simulink model "ECmodel1"  (R2014a)
settings: Solver=ode3  StartTime=0.0  StopTime=6000  FixedStep=10  MaxStep=10  MinStep=10  RelTol=1e-3
settings Model: Creator=Suda  LastModifiedBy=杰

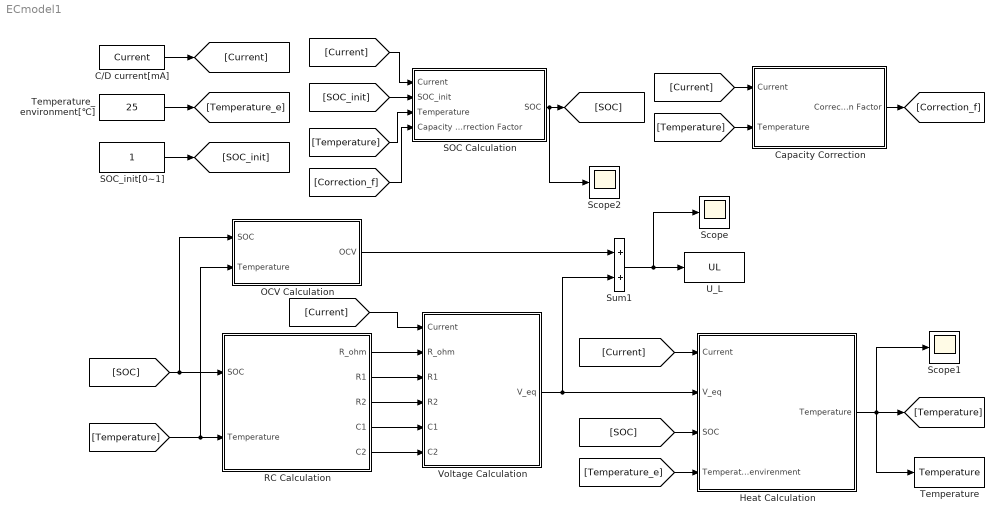
== system ECmodel1 ==
  C/D current[mA] : FromWorkspace  VariableName=Current  SampleTime=0
  Capacity Correction : Subsystem
  Heat Calculation : Subsystem
  OCV Calculation : Subsystem
  RC Calculation : Subsystem
  SOC Calculation : Subsystem
  SOC_init[0~1] : Constant
  Scope : Scope
  Scope1 : Scope
  Scope2 : Scope
      settings: SaveName=ScopeData2
  Sum1 : Sum
  Temperature : ToWorkspace  VariableName=Temperature  SaveFormat=Structure With Time  SampleTime=-1
  Temperature_environment[℃] : Constant  Value=25
  U_L : ToWorkspace  VariableName=UL  SaveFormat=Structure With Time  SampleTime=-1
  Voltage Calculation : Subsystem
  wires:
  OCV Calculation/1(OCV) -> Sum1/1
  RC Calculation/1(R_ohm) -> Voltage Calculation/2("R_ohm ")
  RC Calculation/2(R1) -> Voltage Calculation/3(R1)
  RC Calculation/3(R2) -> Voltage Calculation/4(R2)
  RC Calculation/4(C1) -> Voltage Calculation/5(C1)
  RC Calculation/5(C2) -> Voltage Calculation/6(C2)
  Voltage Calculation/1(V_eq) -> Heat Calculation/2(V_eq), Sum1/2
  Sum1/1 -> Scope/1, U_L/1
  C/D current[mA]/1 -> [Current]
  [Current] -> SOC Calculation/1(Current)
  Temperature_environment[℃]/1 -> [Temperature_e]
  [Temperature] -> SOC Calculation/3("Temperature ")
  SOC Calculation/1(SOC) -> Scope2/1, [SOC]
  [Temperature] -> OCV Calculation/2(Temperature), RC Calculation/2(Temperature)
  [Current] -> Voltage Calculation/1(Current)
  [SOC] -> RC Calculation/1(SOC), OCV Calculation/1(SOC)
  SOC_init[0~1]/1 -> [SOC_init]
  [SOC_init] -> SOC Calculation/2(SOC_init)
  [Temperature_e] -> Heat Calculation/4(Temperature_envirenment)
  [Current] -> Heat Calculation/1(Current)
  Heat Calculation/1(Temperature) -> Temperature/1, Scope1/1, [Temperature]
  [SOC] -> Heat Calculation/3(SOC)
  [Current] -> Capacity Correction/1(Current)
  [Temperature] -> Capacity Correction/2(Temperature)
  [Correction_f] -> SOC Calculation/4(Capacity Correction Factor)
  Capacity Correction/1(" Correction Factor") -> [Correction_f]

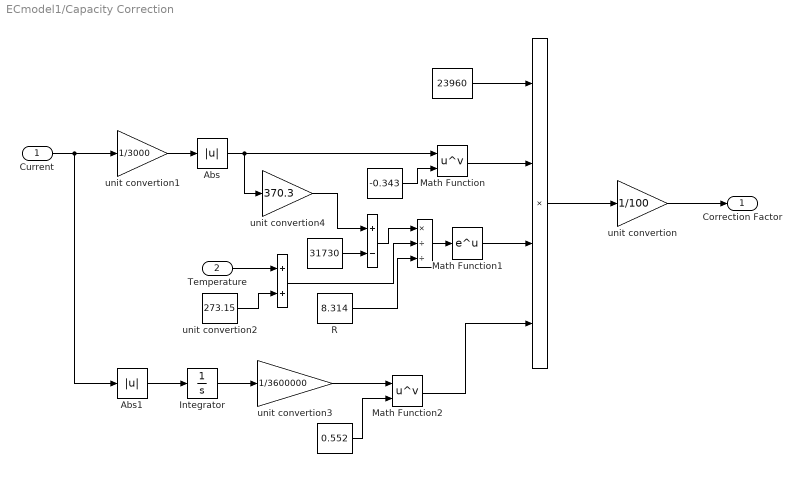
== system ECmodel1/Capacity Correction ==
  Current : Inport
  Temperature : Inport  Port=2
  "  " : Product  Inputs=4
  "     " : Constant  Value=-0.343
  "      " : Constant  Value=23960
  "       " : Constant  Value=31730
  "         " : Sum  Inputs=+-
  "            " : Product  Inputs=*//
  "              " : Sum
  "                 " : Constant  Value=0.552
  Abs : Abs
  Abs1 : Abs
  Integrator : Integrator
  Math Function : Math  Operator=pow  SaturateOnIntegerOverflow=on
  Math Function1 : Math  SaturateOnIntegerOverflow=on
  Math Function2 : Math  Operator=pow  SaturateOnIntegerOverflow=on
  R : Constant  Value=8.314
  unit convertion : Gain  Gain=1/100
  unit convertion1 : Gain  Gain=1/3000
  unit convertion2 : Constant  Value=273.15
  unit convertion3 : Gain  Gain=1/3600000
  unit convertion4 : Gain  Gain=370.3
  " Correction Factor" : Outport
  wires:
  Current/1 -> Abs1/1, unit convertion1/1
  unit convertion1/1 -> Abs/1
  "  "/1 -> unit convertion/1
  "      "/1 -> "  "/1
  Abs/1 -> unit convertion4/1, Math Function/1
  "     "/1 -> Math Function/2
  Math Function/1 -> "  "/2
  Temperature/1 -> "              "/1
  unit convertion2/1 -> "              "/2
  "         "/1 -> "            "/1
  "              "/1 -> "            "/2
  R/1 -> "            "/3
  "            "/1 -> Math Function1/1
  Math Function1/1 -> "  "/3
  Abs1/1 -> Integrator/1
  Integrator/1 -> unit convertion3/1
  "                 "/1 -> Math Function2/2
  Math Function2/1 -> "  "/4
  unit convertion4/1 -> "         "/1
  "       "/1 -> "         "/2
  unit convertion/1 -> " Correction Factor"/1
  unit convertion3/1 -> Math Function2/1

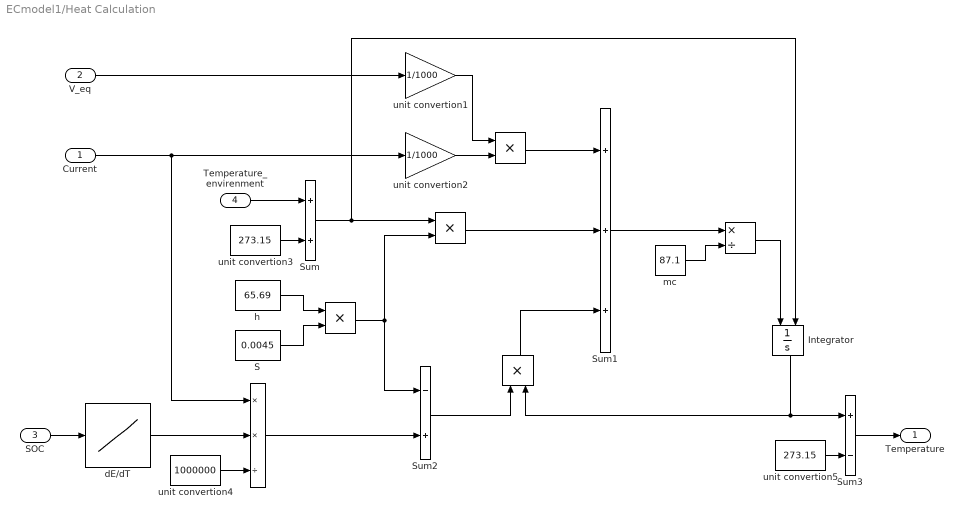
== system ECmodel1/Heat Calculation ==
  Current : Inport
  V_eq : Inport  Port=2
  SOC : Inport  Port=3
  Temperature_envirenment : Inport  Port=4
  "    " : Product
  "     " : Product
  "      " : Product  Inputs=**/
  "       " : Product
  "        " : Product  Inputs=*/
  "                 " : Product
  Integrator : Integrator  InitialConditionSource=external  InitialCondition=273.15
  S : Constant  Value=0.0045
  Sum : Sum
  Sum1 : Sum  Inputs=+++
  Sum2 : Sum  Inputs=-+
  Sum3 : Sum  Inputs=+-
  dE/dT : Lookup_n-D  NumberOfTableDimensions=1  BreakpointsForDimension1=[0.0017,0.0922,0.1907,0.2864,0.3863,0.4883,0.5783,0.6797,0.7686,0.8744,0.9685]  Table=[-0.2986,-0.2442,-0.1088,-0.0392,0.0456,0.0709,0.1089,0.1152,0.0482,0.057,0.1331]  InternalRulePriority=Speed  RndMeth=Simplest  InputSameDT=on
  h : Constant  Value=65.69
  mc : Constant  Value=87.1
  unit convertion1 : Gain  Gain=1/1000
  unit convertion2 : Gain  Gain=1/1000
  unit convertion3 : Constant  Value=273.15
  unit convertion4 : Constant  Value=1000000
  unit convertion5 : Constant  Value=273.15
  Temperature : Outport
  wires:
  V_eq/1 -> unit convertion1/1
  Current/1 -> unit convertion2/1, "      "/1
  unit convertion1/1 -> "    "/1
  unit convertion2/1 -> "    "/2
  Temperature_envirenment/1 -> Sum/1
  unit convertion3/1 -> Sum/2
  h/1 -> "     "/1
  S/1 -> "     "/2
  Sum/1 -> Integrator/2, "       "/1
  "     "/1 -> Sum2/1, "       "/2
  SOC/1 -> dE/dT/1
  dE/dT/1 -> "      "/2
  unit convertion4/1 -> "      "/3
  "      "/1 -> Sum2/2
  unit convertion5/1 -> Sum3/2
  "    "/1 -> Sum1/1
  "       "/1 -> Sum1/2
  Sum2/1 -> "                 "/1
  "                 "/1 -> Sum1/3
  Sum1/1 -> "        "/1
  mc/1 -> "        "/2
  "        "/1 -> Integrator/1
  Integrator/1 -> "                 "/2, Sum3/1
  Sum3/1 -> Temperature/1

== system ECmodel1/OCV Calculation ==
  SOC : Inport
  Temperature : Inport  Port=2
  -10℃ : Subsystem
  10℃ : Subsystem
  25℃ : Subsystem
  40℃ : Subsystem
  55℃ : Subsystem
  Chart : Stateflow chart  TreatAsAtomicUnit=on
  OCV : Outport
  wires:
  SOC/1 -> 55℃/1(SOC), 40℃/1(SOC), 25℃/1(SOC), 10℃/1(SOC), -10℃/1(SOC)
  Temperature/1 -> Chart/1(T)
  -10℃/1(OCV_-10) -> Chart/2(OCV_N10)
  10℃/1(OCV_10) -> Chart/3(OCV_10)
  25℃/1(OCV_25) -> Chart/4(OCV_25)
  40℃/1(OCV_40) -> Chart/5(OCV_40)
  55℃/1(OCV_55) -> Chart/6(OCV_55)
  Chart/1(OCV) -> OCV/1

== system ECmodel1/RC Calculation ==
  SOC : Inport
  Temperature : Inport  Port=2
  Subsystem : Subsystem
  Subsystem1 : Subsystem
  Subsystem2 : Subsystem
  Subsystem3 : Subsystem
  Subsystem4 : Subsystem
  R_ohm : Outport
  R1 : Outport  Port=2
  R2 : Outport  Port=3
  C1 : Outport  Port=4
  C2 : Outport  Port=5
  wires:
  Temperature/1 -> Subsystem4/1(Tempearture), Subsystem3/1(Temperature), Subsystem2/1(Temperature), Subsystem1/1(Tempearture), Subsystem/2(Temperature)
  Subsystem/1(R_ohm) -> R_ohm/1
  Subsystem1/1(R1) -> R1/1
  Subsystem2/1(C1) -> C1/1
  Subsystem3/1(R2) -> R2/1
  Subsystem4/1(C2) -> C2/1
  SOC/1 -> Subsystem/1(SOC)

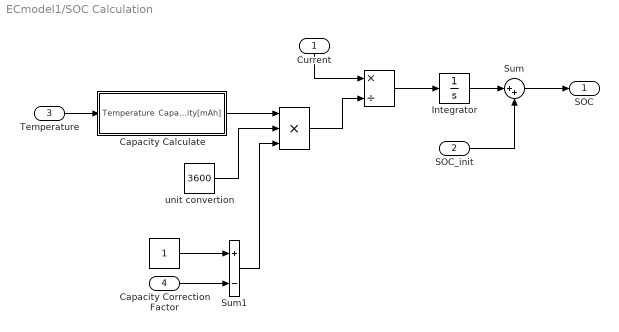
== system ECmodel1/SOC Calculation ==
  Current : Inport
  SOC_init : Inport  Port=2
  "Temperature " : Inport  Port=3
  Capacity Correction Factor : Inport  Port=4
  " " : Constant
  "  " : Product  Inputs=*/
  "    " : Product  Inputs=3
  Capacity Calculate : Subsystem
  Integrator : Integrator
  Sum : Sum  Inputs=|++
  Sum1 : Sum  Inputs=+-
  unit convertion : Constant  Value=3600
  SOC : Outport
  wires:
  "Temperature "/1 -> Capacity Calculate/1(Temperature)
  "    "/1 -> "  "/2
  Integrator/1 -> Sum/1
  SOC_init/1 -> Sum/2
  "  "/1 -> Integrator/1
  Current/1 -> "  "/1
  Capacity Calculate/1(Capacity[mAh]) -> "    "/1
  unit convertion/1 -> "    "/2
  Sum/1 -> SOC/1
  " "/1 -> Sum1/1
  Capacity Correction Factor/1 -> Sum1/2
  Sum1/1 -> "    "/3

== system ECmodel1/Voltage Calculation ==
  Current : Inport
  "R_ohm " : Inport  Port=2
  R1 : Inport  Port=3
  R2 : Inport  Port=4
  C1 : Inport  Port=5
  C2 : Inport  Port=6
  Product : Product
  Subsystem : Subsystem
  Subsystem1 : Subsystem
  Sum : Sum  Inputs=+++
  V_eq : Outport
  wires:
  "R_ohm "/1 -> Product/1
  Product/1 -> Sum/1
  Sum/1 -> V_eq/1
  Current/1 -> Subsystem1/2(Current), Subsystem/2(Current), Product/2
  C1/1 -> Subsystem/1(C1)
  R1/1 -> Subsystem/3(R1)
  Subsystem/1(V1) -> Sum/2
  C2/1 -> Subsystem1/1(C2)
  R2/1 -> Subsystem1/3(R2)
  Subsystem1/1(V2) -> Sum/3

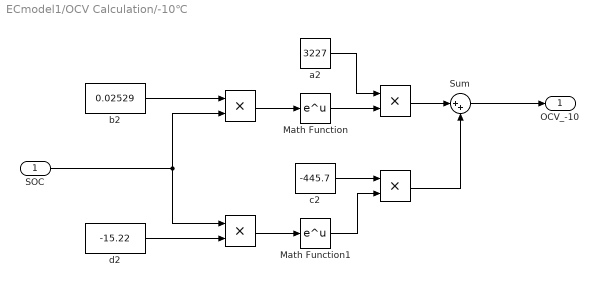
== system ECmodel1/OCV Calculation/-10℃ ==
  SOC : Inport
  " " : Product
  "  " : Product
  "   " : Product
  "    " : Product
  Math Function : Math  SaturateOnIntegerOverflow=on
  Math Function1 : Math  SaturateOnIntegerOverflow=on
  Sum : Sum  Inputs=|++
  a2 : Constant  Value=3227
  b2 : Constant  Value=0.02529
  c2 : Constant  Value=-445.7
  d2 : Constant  Value=-15.22
  OCV_-10 : Outport
  wires:
  Sum/1 -> OCV_-10/1
  d2/1 -> "  "/2
  SOC/1 -> " "/2, "  "/1
  " "/1 -> Math Function/1
  Math Function1/1 -> "    "/2
  "  "/1 -> Math Function1/1
  Math Function/1 -> "   "/2
  c2/1 -> "    "/1
  "   "/1 -> Sum/1
  "    "/1 -> Sum/2
  b2/1 -> " "/1
  a2/1 -> "   "/1

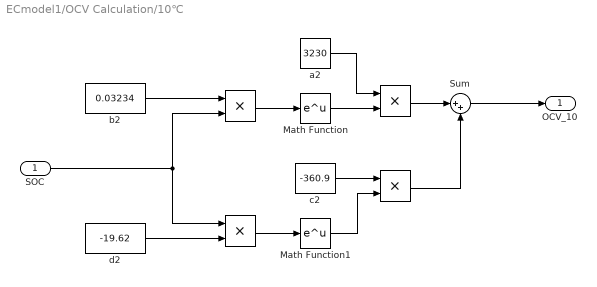
== system ECmodel1/OCV Calculation/10℃ ==
  SOC : Inport
  " " : Product
  "  " : Product
  "   " : Product
  "    " : Product
  Math Function : Math  SaturateOnIntegerOverflow=on
  Math Function1 : Math  SaturateOnIntegerOverflow=on
  Sum : Sum  Inputs=|++
  a2 : Constant  Value=3230
  b2 : Constant  Value=0.03234
  c2 : Constant  Value=-360.9
  d2 : Constant  Value=-19.62
  OCV_10 : Outport
  wires:
  Sum/1 -> OCV_10/1
  d2/1 -> "  "/2
  SOC/1 -> " "/2, "  "/1
  " "/1 -> Math Function/1
  Math Function1/1 -> "    "/2
  "  "/1 -> Math Function1/1
  Math Function/1 -> "   "/2
  c2/1 -> "    "/1
  "   "/1 -> Sum/1
  "    "/1 -> Sum/2
  b2/1 -> " "/1
  a2/1 -> "   "/1

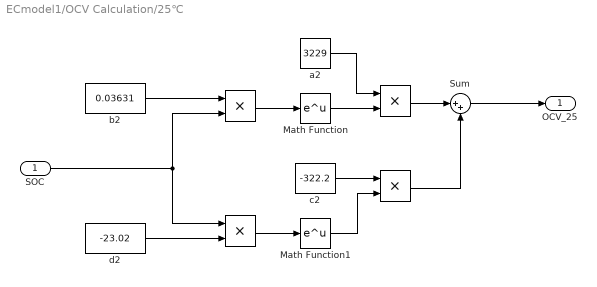
== system ECmodel1/OCV Calculation/25℃ ==
  SOC : Inport
  " " : Product
  "  " : Product
  "   " : Product
  "    " : Product
  Math Function : Math  SaturateOnIntegerOverflow=on
  Math Function1 : Math  SaturateOnIntegerOverflow=on
  Sum : Sum  Inputs=|++
  a2 : Constant  Value=3229
  b2 : Constant  Value=0.03631
  c2 : Constant  Value=-322.2
  d2 : Constant  Value=-23.02
  OCV_25 : Outport
  wires:
  Sum/1 -> OCV_25/1
  d2/1 -> "  "/2
  SOC/1 -> " "/2, "  "/1
  " "/1 -> Math Function/1
  Math Function1/1 -> "    "/2
  "  "/1 -> Math Function1/1
  Math Function/1 -> "   "/2
  c2/1 -> "    "/1
  "   "/1 -> Sum/1
  "    "/1 -> Sum/2
  b2/1 -> " "/1
  a2/1 -> "   "/1

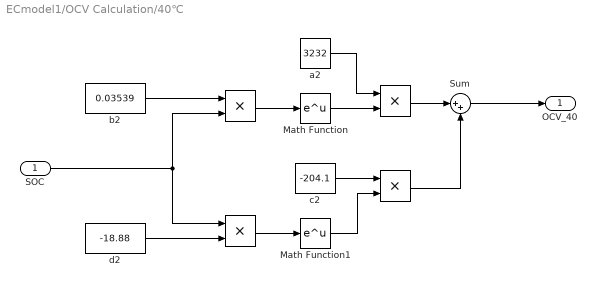
== system ECmodel1/OCV Calculation/40℃ ==
  SOC : Inport
  " " : Product
  "  " : Product
  "   " : Product
  "    " : Product
  Math Function : Math  SaturateOnIntegerOverflow=on
  Math Function1 : Math  SaturateOnIntegerOverflow=on
  Sum : Sum  Inputs=|++
  a2 : Constant  Value=3232
  b2 : Constant  Value=0.03539
  c2 : Constant  Value=-204.1
  d2 : Constant  Value=-18.88
  OCV_40 : Outport
  wires:
  Sum/1 -> OCV_40/1
  d2/1 -> "  "/2
  SOC/1 -> " "/2, "  "/1
  " "/1 -> Math Function/1
  Math Function1/1 -> "    "/2
  "  "/1 -> Math Function1/1
  Math Function/1 -> "   "/2
  c2/1 -> "    "/1
  "   "/1 -> Sum/1
  "    "/1 -> Sum/2
  b2/1 -> " "/1
  a2/1 -> "   "/1

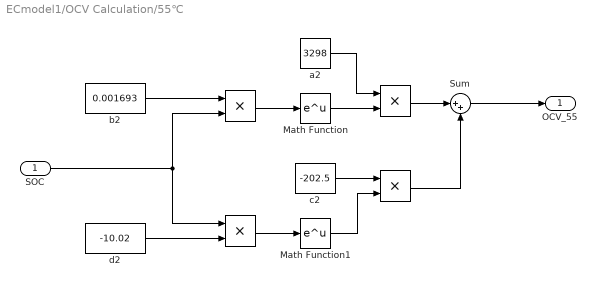
== system ECmodel1/OCV Calculation/55℃ ==
  SOC : Inport
  " " : Product
  "  " : Product
  "   " : Product
  "    " : Product
  Math Function : Math  SaturateOnIntegerOverflow=on
  Math Function1 : Math  SaturateOnIntegerOverflow=on
  Sum : Sum  Inputs=|++
  a2 : Constant  Value=3298
  b2 : Constant  Value=0.001693
  c2 : Constant  Value=-202.5
  d2 : Constant  Value=-10.02
  OCV_55 : Outport
  wires:
  Sum/1 -> OCV_55/1
  d2/1 -> "  "/2
  SOC/1 -> " "/2, "  "/1
  " "/1 -> Math Function/1
  Math Function1/1 -> "    "/2
  "  "/1 -> Math Function1/1
  Math Function/1 -> "   "/2
  c2/1 -> "    "/1
  "   "/1 -> Sum/1
  "    "/1 -> Sum/2
  b2/1 -> " "/1
  a2/1 -> "   "/1

== system ECmodel1/RC Calculation/Subsystem ==
  SOC : Inport
  Temperature : Inport  Port=2
  -10℃ : Subsystem
  10℃ : Subsystem
  25℃ : Subsystem
  40℃ : Subsystem
  55℃ : Subsystem
  Chart : Stateflow chart  TreatAsAtomicUnit=on
  R_ohm : Outport
  wires:
  Temperature/1 -> Chart/1(T)
  -10℃/1(ohm_-10) -> Chart/2(ohm_N10)
  10℃/1(ohm_10) -> Chart/3(ohm_10)
  25℃/1(ohm_25) -> Chart/4(ohm_25)
  40℃/1(ohm_40) -> Chart/5(ohm_40)
  55℃/1(ohm_55) -> Chart/6(ohm_55)
  Chart/1(R_ohm) -> R_ohm/1
  SOC/1 -> 55℃/1(SOC), 40℃/1(SOC), 25℃/1(SOC), 10℃/1(SOC), -10℃/1(SOC)

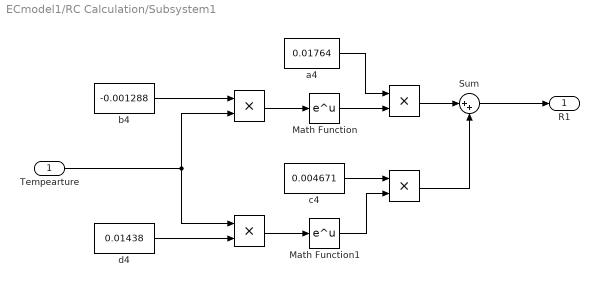
== system ECmodel1/RC Calculation/Subsystem1 ==
  Tempearture : Inport
  " " : Product
  "  " : Product
  "   " : Product
  "    " : Product
  Math Function : Math  SaturateOnIntegerOverflow=on
  Math Function1 : Math  SaturateOnIntegerOverflow=on
  Sum : Sum  Inputs=|++
  a4 : Constant  Value=0.01764
  b4 : Constant  Value=-0.001288
  c4 : Constant  Value=0.004671
  d4 : Constant  Value=0.01438
  R1 : Outport
  wires:
  Sum/1 -> R1/1
  d4/1 -> "  "/2
  Tempearture/1 -> " "/2, "  "/1
  " "/1 -> Math Function/1
  Math Function1/1 -> "    "/2
  "  "/1 -> Math Function1/1
  Math Function/1 -> "   "/2
  c4/1 -> "    "/1
  "   "/1 -> Sum/1
  "    "/1 -> Sum/2
  b4/1 -> " "/1
  a4/1 -> "   "/1

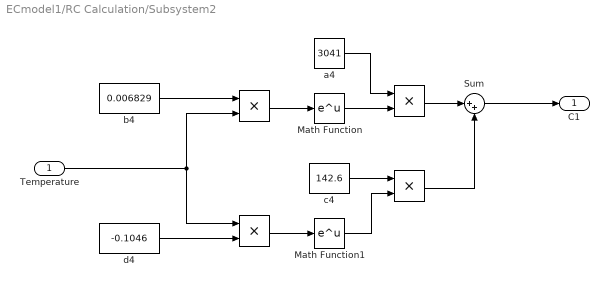
== system ECmodel1/RC Calculation/Subsystem2 ==
  Temperature : Inport
  " " : Product
  "  " : Product
  "   " : Product
  "    " : Product
  Math Function : Math  SaturateOnIntegerOverflow=on
  Math Function1 : Math  SaturateOnIntegerOverflow=on
  Sum : Sum  Inputs=|++
  a4 : Constant  Value=3041
  b4 : Constant  Value=0.006829
  c4 : Constant  Value=142.6
  d4 : Constant  Value=-0.1046
  C1 : Outport
  wires:
  Sum/1 -> C1/1
  d4/1 -> "  "/2
  Temperature/1 -> " "/2, "  "/1
  " "/1 -> Math Function/1
  Math Function1/1 -> "    "/2
  "  "/1 -> Math Function1/1
  Math Function/1 -> "   "/2
  c4/1 -> "    "/1
  "   "/1 -> Sum/1
  "    "/1 -> Sum/2
  b4/1 -> " "/1
  a4/1 -> "   "/1

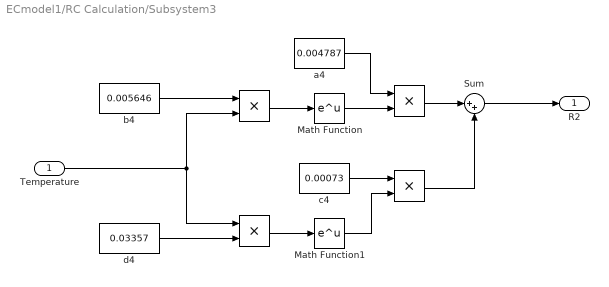
== system ECmodel1/RC Calculation/Subsystem3 ==
  Temperature : Inport
  " " : Product
  "  " : Product
  "   " : Product
  "    " : Product
  Math Function : Math  SaturateOnIntegerOverflow=on
  Math Function1 : Math  SaturateOnIntegerOverflow=on
  Sum : Sum  Inputs=|++
  a4 : Constant  Value=0.004787
  b4 : Constant  Value=0.005646
  c4 : Constant  Value=0.00073
  d4 : Constant  Value=0.03357
  R2 : Outport
  wires:
  Sum/1 -> R2/1
  d4/1 -> "  "/2
  Temperature/1 -> " "/2, "  "/1
  " "/1 -> Math Function/1
  Math Function1/1 -> "    "/2
  "  "/1 -> Math Function1/1
  Math Function/1 -> "   "/2
  c4/1 -> "    "/1
  "   "/1 -> Sum/1
  "    "/1 -> Sum/2
  b4/1 -> " "/1
  a4/1 -> "   "/1

== system ECmodel1/RC Calculation/Subsystem4 ==
  Tempearture : Inport
  " " : Product
  "  " : Product
  "   " : Product
  "    " : Product
  Math Function : Math  SaturateOnIntegerOverflow=on
  Math Function1 : Math  SaturateOnIntegerOverflow=on
  Sum : Sum  Inputs=|++
  a4 : Constant  Value=-5.5e-13
  b4 : Constant  Value=0.6517
  c4 : Constant  Value=26300
  d4 : Constant  Value=-0.005202
  C2 : Outport
  wires:
  Sum/1 -> C2/1
  d4/1 -> "  "/2
  Tempearture/1 -> " "/2, "  "/1
  " "/1 -> Math Function/1
  Math Function1/1 -> "    "/2
  "  "/1 -> Math Function1/1
  Math Function/1 -> "   "/2
  c4/1 -> "    "/1
  "   "/1 -> Sum/1
  "    "/1 -> Sum/2
  b4/1 -> " "/1
  a4/1 -> "   "/1

== system ECmodel1/SOC Calculation/Capacity Calculate ==
  Temperature : Inport
  " " : Product
  "  " : Product
  "   " : Product
  "    " : Product
  Math Function : Math  SaturateOnIntegerOverflow=on
  Math Function1 : Math  SaturateOnIntegerOverflow=on
  Sum : Sum  Inputs=|++
  a1 : Constant  Value=2949
  b1 : Constant  Value=0.001464
  c1 : Constant  Value=-46.07
  d1 : Constant  Value=-0.146
  Capacity[mAh] : Outport
  wires:
  d1/1 -> "  "/2
  Sum/1 -> Capacity[mAh]/1
  Temperature/1 -> " "/2, "  "/1
  "    "/1 -> Sum/2
  b1/1 -> " "/1
  Math Function/1 -> "   "/2
  " "/1 -> Math Function/1
  Math Function1/1 -> "    "/2
  "  "/1 -> Math Function1/1
  c1/1 -> "    "/1
  "   "/1 -> Sum/1
  a1/1 -> "   "/1

== system ECmodel1/Voltage Calculation/Subsystem ==
  C1 : Inport
  Current : Inport  Port=2
  R1 : Inport  Port=3
  " " : Product
  "  " : Product
  Fcn : Fcn  Expr=1/u
  Fcn1 : Fcn  Expr=1/u
  Integrator : Integrator
  Sum1 : Sum  Inputs=|+-
  V1 : Outport
  wires:
  Current/1 -> Sum1/1
  Fcn1/1 -> "  "/2
  "  "/1 -> Sum1/2
  Fcn/1 -> " "/1
  Sum1/1 -> " "/2
  C1/1 -> Fcn/1
  " "/1 -> Integrator/1
  R1/1 -> Fcn1/1
  Integrator/1 -> V1/1, "  "/1

== system ECmodel1/Voltage Calculation/Subsystem1 ==
  C2 : Inport
  Current : Inport  Port=2
  R2 : Inport  Port=3
  " " : Product
  "  " : Product
  Fcn2 : Fcn  Expr=1/u
  Fcn3 : Fcn  Expr=1/u
  Integrator1 : Integrator
  Sum2 : Sum  Inputs=|+-
  V2 : Outport
  wires:
  Current/1 -> Sum2/1
  Sum2/1 -> " "/2
  C2/1 -> Fcn2/1
  Fcn2/1 -> " "/1
  R2/1 -> Fcn3/1
  " "/1 -> Integrator1/1
  Integrator1/1 -> V2/1, "  "/1
  Fcn3/1 -> "  "/2
  "  "/1 -> Sum2/2

== system ECmodel1/RC Calculation/Subsystem/-10℃ ==
  SOC : Inport
  " " : Product
  "  " : Product
  "   " : Product
  "    " : Product
  Math Function : Math  SaturateOnIntegerOverflow=on
  Math Function1 : Math  SaturateOnIntegerOverflow=on
  Sum : Sum  Inputs=|++
  a3 : Constant  Value=-7.382
  b3 : Constant  Value=1.097
  c3 : Constant  Value=8.364
  d3 : Constant  Value=0.9984
  ohm_-10 : Outport
  wires:
  Sum/1 -> ohm_-10/1
  d3/1 -> "  "/2
  SOC/1 -> " "/2, "  "/1
  " "/1 -> Math Function/1
  Math Function1/1 -> "    "/2
  "  "/1 -> Math Function1/1
  Math Function/1 -> "   "/2
  c3/1 -> "    "/1
  "   "/1 -> Sum/1
  "    "/1 -> Sum/2
  b3/1 -> " "/1
  a3/1 -> "   "/1

== system ECmodel1/RC Calculation/Subsystem/10℃ ==
  SOC : Inport
  " " : Product
  "  " : Product
  "   " : Product
  "    " : Product
  Math Function : Math  SaturateOnIntegerOverflow=on
  Math Function1 : Math  SaturateOnIntegerOverflow=on
  Sum : Sum  Inputs=|++
  a3 : Constant  Value=0.1901
  b3 : Constant  Value=-0.4899
  c3 : Constant  Value=0.09331
  d3 : Constant  Value=0.434
  ohm_10 : Outport
  wires:
  Sum/1 -> ohm_10/1
  d3/1 -> "  "/2
  SOC/1 -> " "/2, "  "/1
  " "/1 -> Math Function/1
  Math Function1/1 -> "    "/2
  "  "/1 -> Math Function1/1
  Math Function/1 -> "   "/2
  c3/1 -> "    "/1
  "   "/1 -> Sum/1
  "    "/1 -> Sum/2
  b3/1 -> " "/1
  a3/1 -> "   "/1

== system ECmodel1/RC Calculation/Subsystem/25℃ ==
  SOC : Inport
  " " : Product
  "  " : Product
  "   " : Product
  "    " : Product
  Math Function : Math  SaturateOnIntegerOverflow=on
  Math Function1 : Math  SaturateOnIntegerOverflow=on
  Sum : Sum  Inputs=|++
  a3 : Constant  Value=0.0151
  b3 : Constant  Value=-2.504
  c3 : Constant  Value=0.2302
  d3 : Constant  Value=-0.00124
  ohm_25 : Outport
  wires:
  Sum/1 -> ohm_25/1
  d3/1 -> "  "/2
  SOC/1 -> " "/2, "  "/1
  " "/1 -> Math Function/1
  Math Function1/1 -> "    "/2
  "  "/1 -> Math Function1/1
  Math Function/1 -> "   "/2
  c3/1 -> "    "/1
  "   "/1 -> Sum/1
  "    "/1 -> Sum/2
  b3/1 -> " "/1
  a3/1 -> "   "/1

== system ECmodel1/RC Calculation/Subsystem/40℃ ==
  SOC : Inport
  " " : Product
  "  " : Product
  "   " : Product
  "    " : Product
  Math Function : Math  SaturateOnIntegerOverflow=on
  Math Function1 : Math  SaturateOnIntegerOverflow=on
  Sum : Sum  Inputs=|++
  a3 : Constant  Value=0.008852
  b3 : Constant  Value=-10.72
  c3 : Constant  Value=0.2487
  d3 : Constant  Value=-0.02033
  ohm_40 : Outport
  wires:
  Sum/1 -> ohm_40/1
  d3/1 -> "  "/2
  SOC/1 -> " "/2, "  "/1
  " "/1 -> Math Function/1
  Math Function1/1 -> "    "/2
  "  "/1 -> Math Function1/1
  Math Function/1 -> "   "/2
  c3/1 -> "    "/1
  "   "/1 -> Sum/1
  "    "/1 -> Sum/2
  b3/1 -> " "/1
  a3/1 -> "   "/1

== system ECmodel1/RC Calculation/Subsystem/55℃ ==
  SOC : Inport
  " " : Product
  "  " : Product
  "   " : Product
  "    " : Product
  Math Function : Math  SaturateOnIntegerOverflow=on
  Math Function1 : Math  SaturateOnIntegerOverflow=on
  Sum : Sum  Inputs=|++
  a3 : Constant  Value=0.003233
  b3 : Constant  Value=-3.733
  c3 : Constant  Value=0.297
  d3 : Constant  Value=-0.03979
  ohm_55 : Outport
  wires:
  Sum/1 -> ohm_55/1
  d3/1 -> "  "/2
  SOC/1 -> " "/2, "  "/1
  " "/1 -> Math Function/1
  Math Function1/1 -> "    "/2
  "  "/1 -> Math Function1/1
  Math Function/1 -> "   "/2
  c3/1 -> "    "/1
  "   "/1 -> Sum/1
  "    "/1 -> Sum/2
  b3/1 -> " "/1
  a3/1 -> "   "/1

== stateflow chart ECmodel1/RC Calculation/Subsystem/Chart ==
  (default) -> (junction 14)
  (junction 14) -> (junction 15) [order 1] : [T>10]
  (junction 15) -> (junction 16) [order 1] : [T>25]
  (junction 16) -> (junction 29) [order 1] : [T>40]
  (junction 29) -> (junction 34) [order 1] : [T>55]
  (junction 14) -> (junction 10) [order 2] : {R_ohm=ohm_N10+(ohm_10-ohm_N10)*(T+10)/20}
  (junction 15) -> (junction 18) [order 2] : {R_ohm=ohm_10+(ohm_25-ohm_10)*(T-10)/15}
  (junction 16) -> (junction 19) [order 2] : {R_ohm=ohm_25+(ohm_40-ohm_25)*(T-25)/15}
  (junction 29) -> (junction 30) [order 2] : {R_ohm=ohm_40+(ohm_55-ohm_40)*(T-40)/15}
  (junction 34) -> (junction 36) : {R_ohm=ohm_55+(ohm_55-ohm_40)*(T-55)/15}
  (junction 18) -> (junction 10)
  (junction 19) -> (junction 18)
  (junction 30) -> (junction 19)
  (junction 36) -> (junction 30)
  (junction 10) -> (junction 11)
  data: T input; ohm_N10 input; ohm_10 input; ohm_25 input; ohm_40 input; ohm_55 input; R_ohm output

== stateflow chart ECmodel1/OCV Calculation/Chart ==
  (default) -> (junction 14)
  (junction 14) -> (junction 15) [order 1] : [T>10]
  (junction 15) -> (junction 16) [order 1] : [T>25]
  (junction 16) -> (junction 29) [order 1] : [T>40]
  (junction 29) -> (junction 34) [order 1] : [T>55]
  (junction 14) -> (junction 10) [order 2] : {OCV=OCV_N10+(OCV_10-OCV_N10)*(T+10)/20}
  (junction 15) -> (junction 18) [order 2] : {OCV=OCV_10+(OCV_25-OCV_10)*(T-10)/15}
  (junction 16) -> (junction 19) [order 2] : {OCV=OCV_25+(OCV_40-OCV_25)*(T-25)/15}
  (junction 29) -> (junction 30) [order 2] : {OCV=OCV_40+(OCV_55-OCV_40)*(T-40)/15}
  (junction 34) -> (junction 36) : {OCV=OCV_55+(OCV_55-OCV_40)*(T-55)/15}
  (junction 18) -> (junction 10)
  (junction 19) -> (junction 18)
  (junction 30) -> (junction 19)
  (junction 36) -> (junction 30)
  (junction 10) -> (junction 11)
  data: T input; OCV_N10 input; OCV_10 input; OCV_25 input; OCV_40 input; OCV_55 input; OCV output
